simulink model "untitled3"  (R2020b)
settings: Solver=VariableStepAuto  StartTime=0.0  StopTime=10.0  RelTol=1e-3
undefined symbols (not defined in the file): sigbuilder_block
libraries: simulink x3
settings Model: Creator=HP  LastModifiedBy=HP

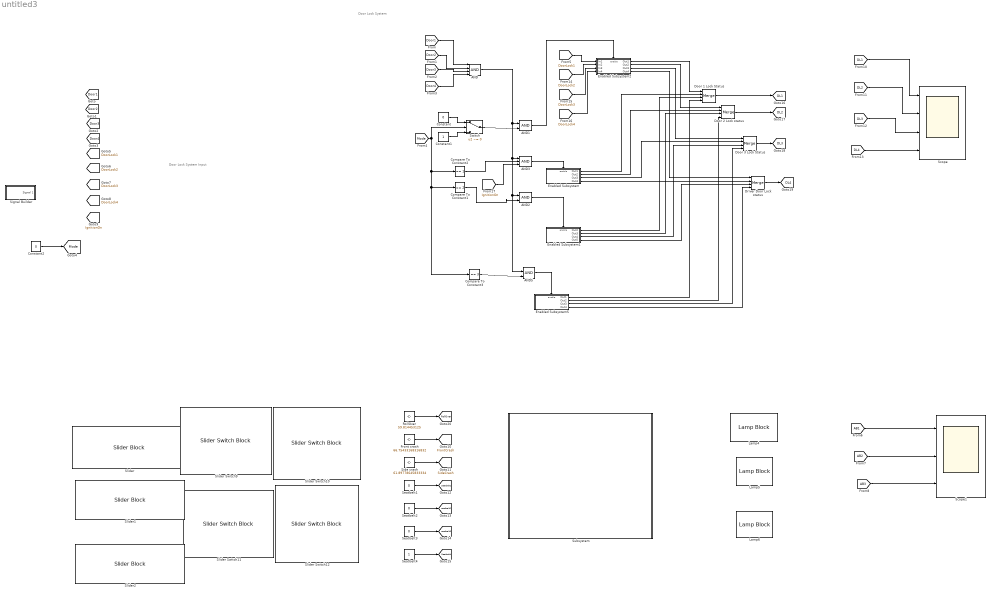
== system untitled3 ==
  note: Door Lock System Input
  note: Door Lock System
  AND : Logic  Inputs=4  IconShape=distinctive  AllPortsSameDT=off  OutDataTypeStr=boolean
  AND1 : Logic  IconShape=distinctive  AllPortsSameDT=off  OutDataTypeStr=boolean
  AND2 : Logic  IconShape=distinctive  AllPortsSameDT=off  OutDataTypeStr=boolean
  AND3 : Logic  Inputs=3  IconShape=distinctive  AllPortsSameDT=off  OutDataTypeStr=boolean
  AND5 : Logic  IconShape=distinctive  AllPortsSameDT=off  OutDataTypeStr=boolean
  Compare To Constant1 : simulink/Logic and Bit Operations/Compare To Constant  relop===  const=2  OutDataTypeStr=boolean
  Compare To Constant2 : simulink/Logic and Bit Operations/Compare To Constant  relop===  const=1  OutDataTypeStr=boolean
  Compare To Constant3 : simulink/Logic and Bit Operations/Compare To Constant  relop===  const=3  OutDataTypeStr=boolean
  Constant : Constant  Value=0
  Constant1 : Constant
  Constant2 : Constant  Value=0
  Door 1 Lock Status : Merge  Inputs=4
  Door 2 Lock status : Merge  Inputs=4
  Door 3 Lock Status : Merge  Inputs=4
  "Driver Door Lock status " : Merge  Inputs=4
  Enabled Subsystem : Subsystem  TreatAsAtomicUnit=on
  Enabled Subsystem1 : Subsystem  TreatAsAtomicUnit=on
  Enabled Subsystem2 : Subsystem  TreatAsAtomicUnit=on
  Enabled Subsystem5 : Subsystem  TreatAsAtomicUnit=on
  Front crash : Constant  Value=66.75433168316832
  Lamp4 : LampBlock
  Lamp5 : LampBlock
  Lamp6 : LampBlock
  RollOver : Constant  Value=59.814453125
  Scope : Scope  NumInputPorts=4
  Scope1 : Scope  NumInputPorts=3
  Seatbelt1 : Constant  Value=0
  Seatbelt2 : Constant  Value=0
  Seatbelt3 : Constant  Value=0
  Seatbelt4 : Constant
  Side crash : Constant  Value=61.89778645833334
  Signal Builder : Subsystem  Tag=STV Subsys  LoadFcn=sigbuilder_block('load');  StartFcn=sigbuilder_block('start');  StopFcn=sigbuilder_block('stop');  ClipboardFcn=sigbuilder_block('clipboard');  mask(Sigbuilder block){tuvar=[0:10]}
      mask help: Simulink:masks:SigbuilderBlock_MD
      mask init:
      | if ~strcmp(get_param(bdroot(gcbh),'SimulationStatus'),'stopped') tuvar = sigbuilder_block('maskInit'); end
      settings: CopyFcn=sigbuilder_block('copy');  DeleteFcn=sigbuilder_block('delete');  ModelCloseFcn=sigbuilder_block('modelClose');  PreSaveFcn=sigbuilder_block('preSave');  PauseFcn=sigbuilder_block('pause');  ContinueFcn=sigbuilder_block('continue');  NameChangeFcn=sigbuilder_block('namechange');  OpenFcn=sigbuilder_block('open',[437.6 199.2 550.4 400 ]);  CloseFcn=sigbuilder_block('close');
      mask Display: plot(0, 0, 100, 100,[2, 2, 32, 32, 2], [68, 8, 8, 68, 68],[32, 2], [38, 38], [32, 19, 2],[53, 60, 44], [32, 17, 17, 2],[16, 16, 31, 31]);txt = getActiveGroup(gcbh);text(2, 100, txt,'verticalAlignment', 'top');
  Slider : SliderBlock
  Slider Switch{9..12} (4 alike) : SliderSwitchBlock
      settings: Values={{'Off', 'On'}, [0 1]}
  Slider1 : SliderBlock
  Slider2 : SliderBlock
  Subsystem : Subsystem
  Switch : Switch  Criteria=u2 ~= 0
  tag scope: DL1=global, DL2=global, DL3=global, DL4=global, Door1=global, Door2=global, Door3=global, Door4=global, DoorLock1=global, DoorLock2=global, DoorLock3=global, DoorLock4=global, FrontCrash=global, IgnitionOn=global, Mode=global, RollOver=global, Seatbelt1=global, Seatbelt4=global, SideCrash=global, seatbelt2=global, seatbelt3=global
  wires:
  [DL3] -> Scope/3
  [AB3] -> Scope1/3
  Seatbelt3/1 -> [seatbelt3]
  [AB2] -> Scope1/2
  [DL2] -> Scope/2
  Front crash/1 -> [FrontCrash]
  Side crash/1 -> [SideCrash]
  Seatbelt1/1 -> [Seatbelt1]
  Seatbelt2/1 -> [seatbelt2]
  [DL1] -> Scope/1
  [DL4] -> Scope/4
  [AB1] -> Scope1/1
  Seatbelt4/1 -> [Seatbelt4]
  Compare To Constant1/1 -> AND2/2
  Compare To Constant2/1 -> AND3/2
  Enabled Subsystem2/3(Out3) -> Door 3 Lock Status/1
  Enabled Subsystem5/1(Out1) -> Door 1 Lock Status/4
  Door 2 Lock status/1 -> [DL2]
  AND3/1 -> Enabled Subsystem/Enable
  Enabled Subsystem/4(Out4) -> "Driver Door Lock status "/2
  Enabled Subsystem5/4(Out4) -> "Driver Door Lock status "/4
  Constant1/1 -> Switch/3
  Switch/1 -> AND1/2
  Enabled Subsystem/3(Out3) -> Door 3 Lock Status/2
  Enabled Subsystem2/4(Out4) -> "Driver Door Lock status "/1
  Compare To Constant3/1 -> AND5/2
  [Mode] -> Switch/2, Compare To Constant2/1, Compare To Constant1/1, Compare To Constant3/1
  AND2/1 -> Enabled Subsystem1/Enable
  [DoorLock2] -> Enabled Subsystem2/2(In2)
  Constant/1 -> Switch/1
  Enabled Subsystem2/1(Out1) -> Door 1 Lock Status/1
  AND5/1 -> Enabled Subsystem5/Enable
  Enabled Subsystem/2(Out2) -> Door 2 Lock status/2
  [DoorLock1] -> Enabled Subsystem2/1(In1)
  Enabled Subsystem1/1(Out2) -> Door 1 Lock Status/3
  [Door3] -> AND/3
  Enabled Subsystem1/4(Out5) -> "Driver Door Lock status "/3
  [Door1] -> AND/1
  [DoorLock3] -> Enabled Subsystem2/3(In3)
  [IgnitionOn] -> AND3/3
  Enabled Subsystem/1(Out1) -> Door 1 Lock Status/2
  Door 3 Lock Status/1 -> [DL3]
  Enabled Subsystem1/2(Out3) -> Door 2 Lock status/3
  AND/1 -> AND5/1, AND2/1, AND3/1, AND1/1
  [Door2] -> AND/2
  Enabled Subsystem5/3(Out3) -> Door 3 Lock Status/4
  Enabled Subsystem5/2(Out2) -> Door 2 Lock status/4
  [DoorLock4] -> Enabled Subsystem2/4(In4)
  [Door4] -> AND/4
  Enabled Subsystem1/3(Out4) -> Door 3 Lock Status/3
  Door 1 Lock Status/1 -> [DL1]
  AND1/1 -> Enabled Subsystem2/Enable
  Enabled Subsystem2/2(Out2) -> Door 2 Lock status/1
  "Driver Door Lock status "/1 -> [DL4]
  Constant2/1 -> [Mode]
  RollOver/1 -> [RollOver]
  ? -> [Door3]
  ? -> [DoorLock1]
  ? -> [DoorLock4]
  ? -> [DoorLock2]
  ? -> [DoorLock3]
  ? -> [Door4]
  ? -> [IgnitionOn]
  ? -> [Door1]
  ? -> [Door2]

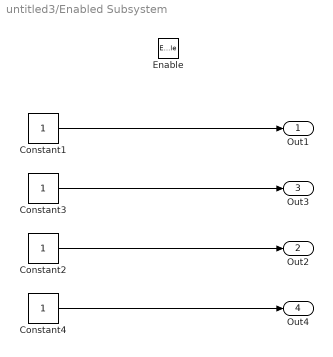
== system untitled3/Enabled Subsystem ==
  Enable : EnablePort
  Constant{1..4} (4 alike) : Constant
  Out1 : Outport
  Out2 : Outport  Port=2
  Out3 : Outport  Port=3
  Out4 : Outport  Port=4
  wires:
  Constant1/1 -> Out1/1
  Constant2/1 -> Out2/1
  Constant3/1 -> Out3/1
  Constant4/1 -> Out4/1

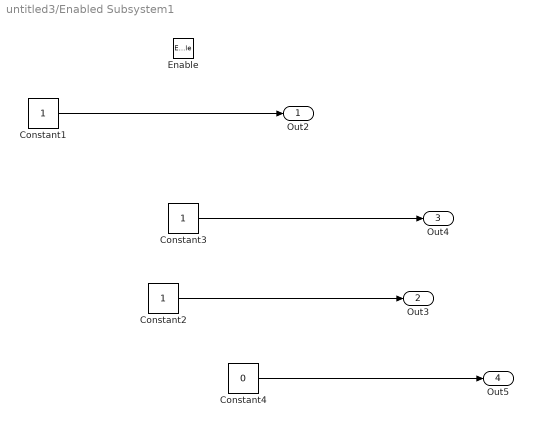
== system untitled3/Enabled Subsystem1 ==
  Enable : EnablePort
  Constant1 : Constant
  Constant2 : Constant
  Constant3 : Constant
  Constant4 : Constant  Value=0
  Out2 : Outport
  Out3 : Outport  Port=2
  Out4 : Outport  Port=3
  Out5 : Outport  Port=4
  wires:
  Constant2/1 -> Out3/1
  Constant3/1 -> Out4/1
  Constant1/1 -> Out2/1
  Constant4/1 -> Out5/1

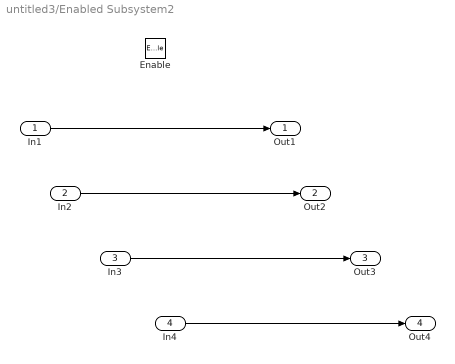
== system untitled3/Enabled Subsystem2 ==
  In1 : Inport
  In2 : Inport  Port=2
  In3 : Inport  Port=3
  In4 : Inport  Port=4
  Enable : EnablePort
  Out1 : Outport
  Out2 : Outport  Port=2
  Out3 : Outport  Port=3
  Out4 : Outport  Port=4
  wires:
  In1/1 -> Out1/1
  In2/1 -> Out2/1
  In3/1 -> Out3/1
  In4/1 -> Out4/1

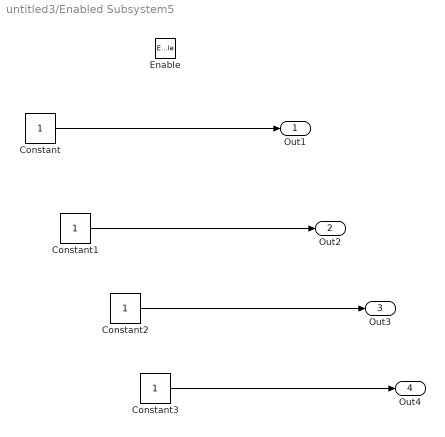
== system untitled3/Enabled Subsystem5 ==
  Enable : EnablePort
  Constant{,1..3} (4 alike) : Constant
  Out1 : Outport
  Out2 : Outport  Port=2
  Out3 : Outport  Port=3
  Out4 : Outport  Port=4
  wires:
  Constant/1 -> Out1/1
  Constant1/1 -> Out2/1
  Constant2/1 -> Out3/1
  Constant3/1 -> Out4/1

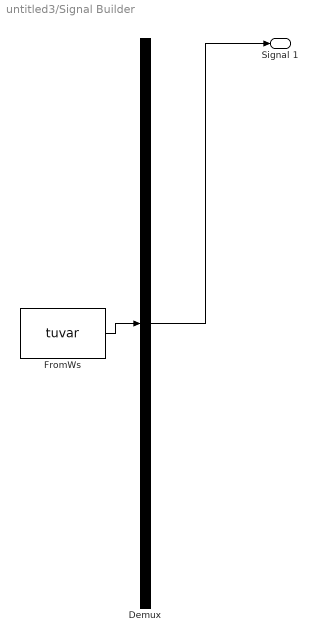
== system untitled3/Signal Builder ==
  Demux : Demux  Tag=STV Demux  Outputs=1
      settings: DisplayOption=none
  FromWs : FromWorkspace  Tag=STV FromWs  VariableName=tuvar
      SigBuilderData=|
      | common.afterFinalStr = 'Extrapolate'
      | common.sampleTime = 0
      | dataSet.timeRange = [0 10]
      | dataSet.name = 'Group 1'
      | sbobj.Groups.Name = 'Group 1'
      | sbobj.Groups.Signals.Name = 'Signal 1'
      | sbobj.Groups.Signals.XData = [0 4 4 6 6 10]
      | sbobj.Groups.Signals.YData = [0 0 1 1 0 0]
  Signal 1 : Outport  Tag=STV Outport
  wires:
  Demux/1 -> Signal 1/1
  FromWs/1 -> Demux/1

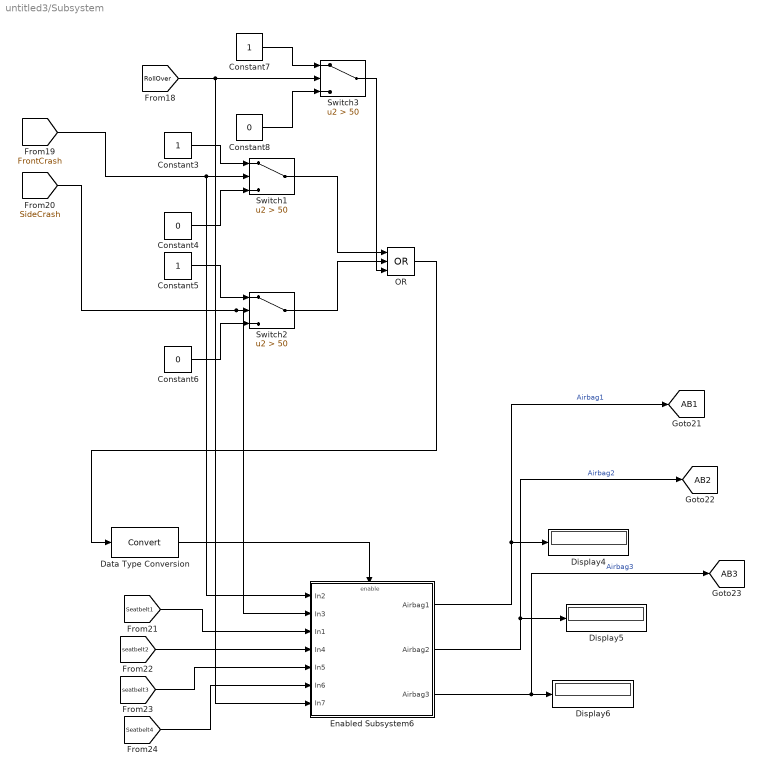
== system untitled3/Subsystem ==
  Constant3 : Constant
  Constant4 : Constant  Value=0
  Constant5 : Constant
  Constant6 : Constant  Value=0
  Constant7 : Constant
  Constant8 : Constant  Value=0
  Data Type Conversion : DataTypeConversion
  Display4 : Display
  Display5 : Display
  Display6 : Display
  Enabled Subsystem6 : Subsystem  TreatAsAtomicUnit=on
  OR : Logic  Operator=OR  Inputs=3  IconShape=distinctive  AllPortsSameDT=off  OutDataTypeStr=boolean
  Switch1 : Switch  Criteria=u2 > Threshold  Threshold=50
  Switch2 : Switch  Criteria=u2 > Threshold  Threshold=50
  Switch3 : Switch  Criteria=u2 > Threshold  Threshold=50
  tag scope: AB1=global, AB2=global, AB3=global
  wires:
  Enabled Subsystem6/2(Airbag2) -> [AB2], Display5/1  "Airbag2"
  Constant7/1 -> Switch3/1
  [Seatbelt4] -> Enabled Subsystem6/6(In6)
  Enabled Subsystem6/3(Airbag3) -> [AB3], Display6/1  "Airbag3"
  [RollOver] -> Enabled Subsystem6/7(In7), Switch3/2
  [seatbelt3] -> Enabled Subsystem6/5(In5)
  [SideCrash] -> Enabled Subsystem6/2(In3), Switch2/2
  Enabled Subsystem6/1(Airbag1) -> [AB1], Display4/1  "Airbag1"
  Data Type Conversion/1 -> Enabled Subsystem6/Enable
  [Seatbelt1] -> Enabled Subsystem6/3(In1)
  Switch3/1 -> OR/3
  Constant5/1 -> Switch2/1
  OR/1 -> Data Type Conversion/1
  Switch1/1 -> OR/1
  Constant6/1 -> Switch2/3
  [FrontCrash] -> Enabled Subsystem6/1(In2), Switch1/2
  Constant8/1 -> Switch3/3
  Switch2/1 -> OR/2
  [seatbelt2] -> Enabled Subsystem6/4(In4)
  Constant3/1 -> Switch1/1
  Constant4/1 -> Switch1/3

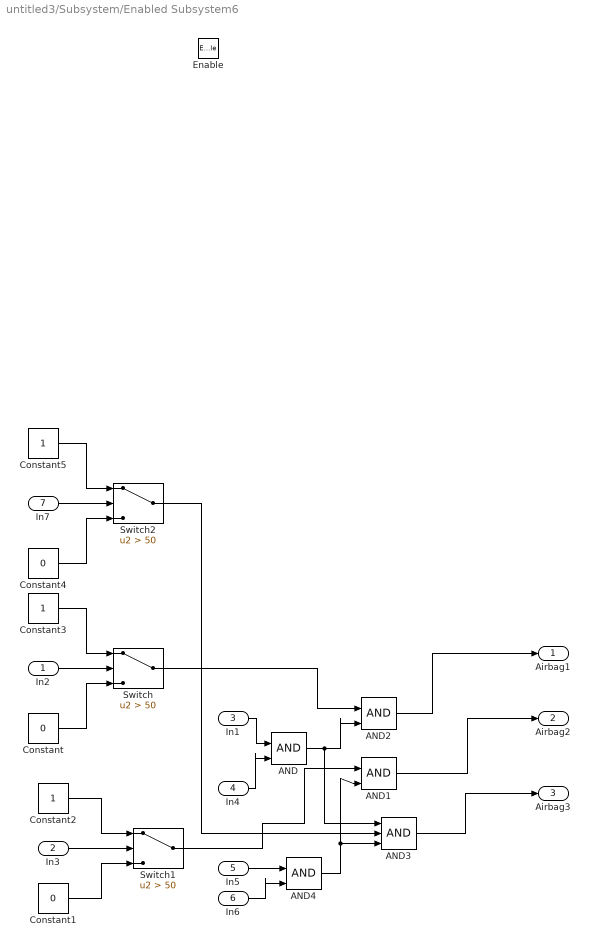
== system untitled3/Subsystem/Enabled Subsystem6 ==
  In2 : Inport
  In3 : Inport  Port=2
  In1 : Inport  Port=3
  In4 : Inport  Port=4
  In5 : Inport  Port=5
  In6 : Inport  Port=6
  In7 : Inport  Port=7
  Enable : EnablePort
  AND{,1..2,4} (4 alike) : Logic  IconShape=distinctive  AllPortsSameDT=off  OutDataTypeStr=boolean
  AND3 : Logic  Inputs=3  IconShape=distinctive  AllPortsSameDT=off  OutDataTypeStr=boolean
  Constant : Constant  Value=0
  Constant1 : Constant  Value=0
  Constant2 : Constant
  Constant3 : Constant
  Constant4 : Constant  Value=0
  Constant5 : Constant
  Switch : Switch  Criteria=u2 > Threshold  Threshold=50
  Switch1 : Switch  Criteria=u2 > Threshold  Threshold=50
  Switch2 : Switch  Criteria=u2 > Threshold  Threshold=50
  Airbag1 : Outport
  Airbag2 : Outport  Port=2
  Airbag3 : Outport  Port=3
  wires:
  Constant2/1 -> Switch1/1
  In2/1 -> Switch/2
  Constant/1 -> Switch/3
  In3/1 -> Switch1/2
  Constant1/1 -> Switch1/3
  Constant3/1 -> Switch/1
  Switch/1 -> AND2/1
  AND2/1 -> Airbag1/1
  AND1/1 -> Airbag2/1
  AND3/1 -> Airbag3/1
  Switch1/1 -> AND1/1
  In1/1 -> AND/1
  In4/1 -> AND/2
  AND/1 -> AND3/1, AND2/2
  In5/1 -> AND4/1
  In6/1 -> AND4/2
  AND4/1 -> AND3/3, AND1/2
  In7/1 -> Switch2/2
  Constant4/1 -> Switch2/3
  Constant5/1 -> Switch2/1
  Switch2/1 -> AND3/2
